simulink model "motorcycle_pole_placement_with_integral_action"  (R2021a)
settings: Solver=VariableStepAuto  StartTime=0.0  StopTime=10  RelTol=1e-3
values from neighbouring files (symbols this model uses):
  A = [0 0;1 0]    [pole_placement.m]
  B = [1; 0]    [pole_placement.m]
  C = [0 1]    [pole_placement.m]
  k = place(A,B,P)    [pole_placement.m]
undefined symbols (not defined in the file or in its folder): L
settings Model: Creator=martina.elle  LastModifiedBy=francesco

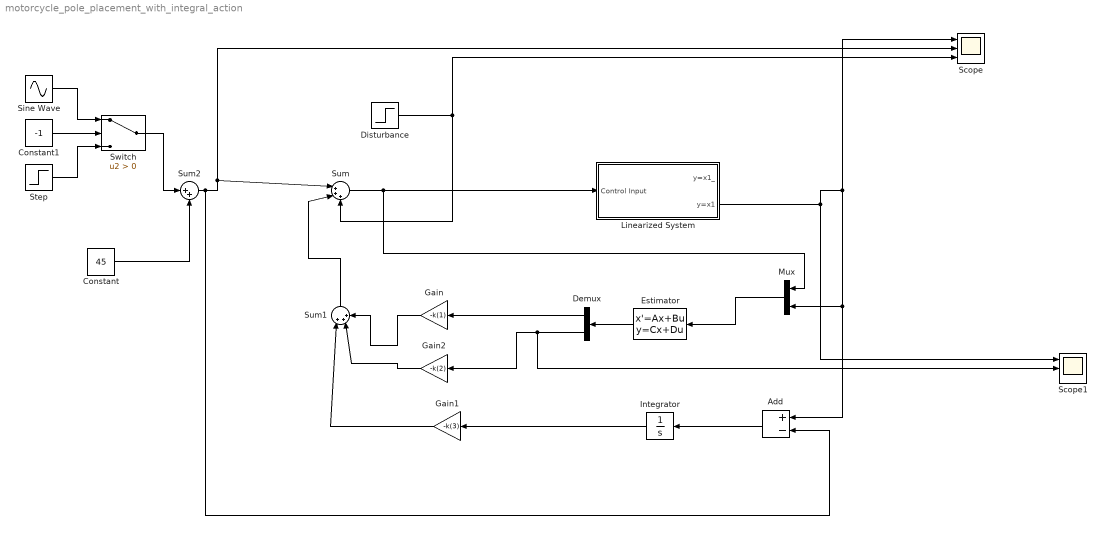
== system motorcycle_pole_placement_with_integral_action ==
  Add : Sum  Inputs=+-
  Constant : Constant  Value=45
  Constant1 : Constant  Value=-1
  Demux : Demux  Outputs=2
  Disturbance : Step  After=3  SampleTime=0
  Estimator : StateSpace  A=A-L*C  B=[B L]  C=eye(2)  D=[0 0; 0 0]  InitialCondition=[10 10]  ParameterTunability=Unconstrained
  Gain : Gain  Gain=-k(1)
  Gain1 : Gain  Gain=-k(3)
  Gain2 : Gain  Gain=-k(2)
  Integrator : Integrator
  Linearized System : Subsystem
  Mux : Mux  Inputs=2
  Scope : Scope  NumInputPorts=3
  Scope1 : Scope  NumInputPorts=3
  Sine Wave : Sin  Frequency=0.1  SampleTime=0
  Step : Step  After=10  SampleTime=0
  Sum : Sum  Inputs=|+++
  Sum1 : Sum  Inputs=|+++
  Sum2 : Sum  Inputs=|++
  Switch : Switch  Criteria=u2 > Threshold
  wires:
  Linearized System/2(y=x1) -> Scope/1, Add/1, Mux/2, Scope1/1
  Sum2/1 -> Add/2, Scope/2, Sum/1
  Sum/1 -> Linearized System/1(Control Input), Mux/1
  Mux/1 -> Estimator/1
  Estimator/1 -> Demux/1
  Demux/1 -> Gain/1
  Gain/1 -> Sum1/3
  Demux/2 -> Scope1/2, Gain2/1
  Gain2/1 -> Sum1/2
  Sum1/1 -> Sum/2
  Switch/1 -> Sum2/1
  Constant/1 -> Sum2/2
  Constant1/1 -> Switch/2
  Sine Wave/1 -> Switch/1
  Step/1 -> Switch/3
  Gain1/1 -> Sum1/1
  Add/1 -> Integrator/1
  Integrator/1 -> Gain1/1
  Disturbance/1 -> Scope/3, Sum/3

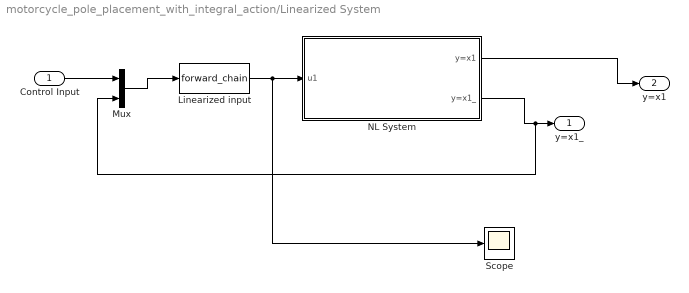
== system motorcycle_pole_placement_with_integral_action/Linearized System ==
  Control Input : Inport
  "Linearized input " : MATLABFcn  MATLABFcn=forward_chain  OutputDimensions=1
  Mux : Mux  Inputs=2
  NL System : Subsystem
  Scope : Scope
  y=x1_ : Outport
  y=x1 : Outport  Port=2
  wires:
  "Linearized input "/1 -> Scope/1, NL System/1(u1)
  NL System/2(y=x1_) -> Mux/2, y=x1_/1
  NL System/1(y=x1) -> y=x1/1
  Control Input/1 -> Mux/1
  Mux/1 -> "Linearized input "/1

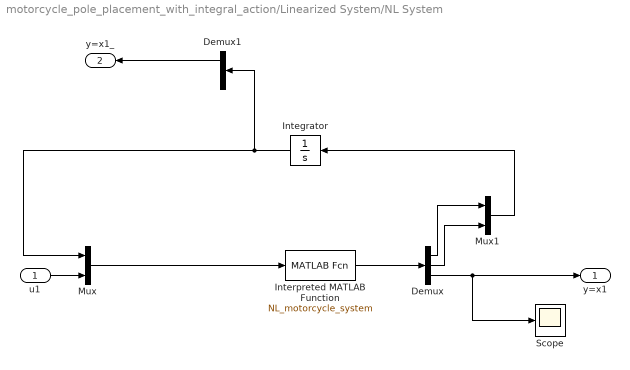
== system motorcycle_pole_placement_with_integral_action/Linearized System/NL System ==
  u1 : Inport
  Demux : Demux  Outputs=3
  Demux1 : Demux  Outputs=2
  Integrator : Integrator  InitialCondition=[5 0]
  Interpreted MATLAB Function : MATLABFcn  MATLABFcn=NL_motorcycle_system  OutputDimensions=3
  Mux : Mux  Inputs=2
  Mux1 : Mux  Inputs=2
  Scope : Scope
  y=x1 : Outport
  y=x1_ : Outport  Port=2
  wires:
  u1/1 -> Mux/2
  Demux/2 -> Mux1/2
  Mux/1 -> Interpreted MATLAB Function/1
  Mux1/1 -> Integrator/1
  Integrator/1 -> Demux1/1, Mux/1
  Demux/1 -> Mux1/1
  Interpreted MATLAB Function/1 -> Demux/1
  Demux/3 -> Scope/1, y=x1/1
  Demux1/1 -> y=x1_/1
